simulink model "controllerDevelopment_Simulink"  (R2020b)
settings: Solver=VariableStepAuto  StartTime=0.0  StopTime=10.0  RelTol=1e-3
undefined symbols (not defined in the file or in its folder): K_PID, x_c_0
libraries: cstblocks x6, pid_lib x1
settings Model: Creator=prenk  LastModifiedBy=prenk

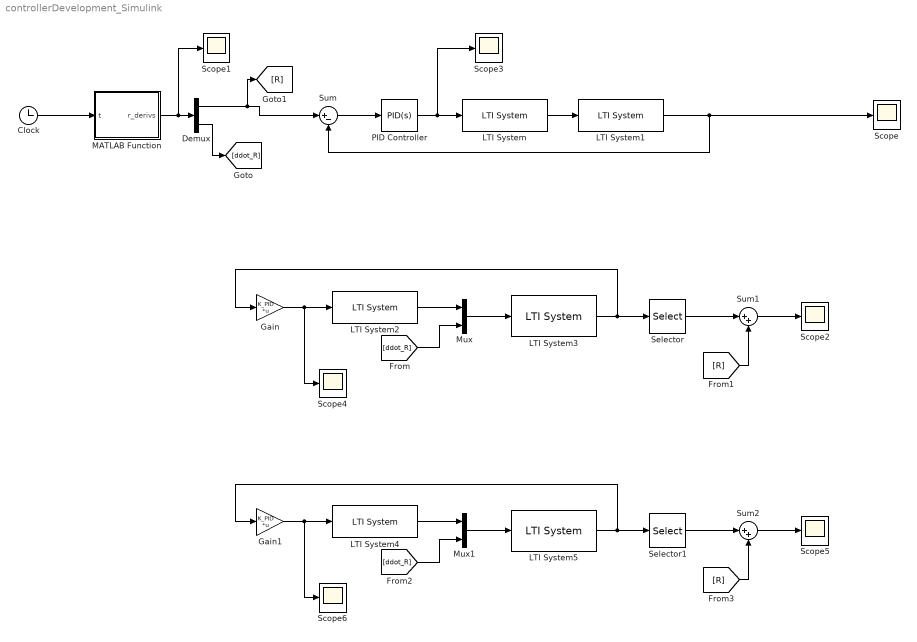
== system controllerDevelopment_Simulink ==
  Clock : Clock
  Demux : Demux  Outputs=2
  Gain : Gain  Gain=K_PID  Multiplication=Matrix(K*u)
  Gain1 : Gain  Gain=K_PID  Multiplication=Matrix(K*u)
  LTI System : cstblocks/LTI System  sys=ssMod_simple_ss  IC=[]
  LTI System1 : cstblocks/LTI System  sys=body  IC=[]
  LTI System2 : cstblocks/LTI System  sys=ssMod_simple_ss  IC=[]
  LTI System3 : cstblocks/LTI System  sys=C_ss  IC=x_c_0
  LTI System4 : cstblocks/LTI System  sys=ssMod_simple_ss  IC=[]
  LTI System5 : cstblocks/LTI System  sys=C_ss  IC=x_c_0
  MATLAB Function : MATLAB Function  TreatAsAtomicUnit=on
  Mux : Mux  Inputs=2
  Mux1 : Mux  Inputs=2
  PID Controller : pid_lib/PID Controller  Controller=PID  Form=Parallel  TimeDomain=Continuous-time  UseExternalTs=off  SampleTime=-1  IntegratorMethod=Forward Euler  FilterMethod=Forward Euler  ControllerParametersSource=internal  P=K_PID(1)  I=K_PID(2)  D=K_PID(3)  UseFilter=on  N=100  TunerSelectOption=Transfer Function Based (PID Tuner App)  InitialConditionSource=internal  InitialConditionForIntegrator=0  InitialConditionForFilter=x_c_0(3)  DifferentiatorICPrevScaledInput=0  ExternalReset=none  TrackingMode=off  Kt=1  LimitOutput=off  SatLimitsSource=internal  UpperSaturationLimit=inf  LowerSaturationLimit=-inf  LinearizeAsGain=on  AntiWindupMode=none  Kb=1  POutMin=[]  POutMax=[]  IOutMin=[]  IOutMax=[]  DOutMin=[]  DOutMax=[]  NOutMin=[]  NOutMax=[]  SumOutMin=[]  SumOutMax=[]  SaturationOutMin=[]  SaturationOutMax=[]  PParamMin=[]  PParamMax=[]  IParamMin=[]  IParamMax=[]  DParamMin=[]  DParamMax=[]  NParamMin=[]  NParamMax=[]  KbParamMin=[]  KbParamMax=[]  KtParamMin=[]  KtParamMax=[]  KbOutMin=[]  KbOutMax=[]  KtOutMin=[]  KtOutMax=[]  IntegratorOutMin=[]  IntegratorOutMax=[]  FilterOutMin=[]  FilterOutMax=[]  SumI1OutMin=[]  SumI1OutMax=[]  SumI2OutMin=[]  SumI2OutMax=[]  SumI3OutMin=[]  SumI3OutMax=[]  SumI4OutMin=[]  SumI4OutMax=[]  SumDOutMin=[]  SumDOutMax=[]  DifferentiatorOutMin=[]  DifferentiatorOutMax=[]  FilterDiffOutCoefMin=[]  FilterDiffOutCoefMax=[]  ReciprocalOutMin=[]  ReciprocalOutMax=[]  SumDenOutMin=[]  SumDenOutMax=[]  SumNumOutMin=[]  SumNumOutMax=[]  DivideOutMin=[]  DivideOutMax=[]  UdiffTsProdOutMin=[]  UdiffTsProdOutMax=[]  NTsProdOutMin=[]  NTsProdOutMax=[]  UintegralTsProdOutMin=[]  UintegralTsProdOutMax=[]  UngainTsProdOutMin=[]  UngainTsProdOutMax=[]  IntegratorContinuousStateAttributes=''  IntegratorStateMustResolveToSignalObject=off  IntegratorRTWStateStorageClass=Auto  FilterContinuousStateAttributes=''  FilterStateMustResolveToSignalObject=off  FilterRTWStateStorageClass=Auto  ParallelPVariant=InternalParameters  IdealPVariant=Disabled  IVariant=InternalParameters  DVariant=InternalParameters  IntegratorVariant=Continuous  SatVariant=Disabled  AWVariant=Passthrough  PCopyVariant=Disabled  TRVariant=Disabled  FdbkBlocksVariant=Forward  IdealPFdbkVariant=Disabled  SatFdbkVariant=Disabled  DerivativeFilterVariant=ContFilter  NVariant=InternalParameters  NCopyVariant=Disabled  FilterICVariant=InternalICsFilter  IntegratorICVariant=InternalICs  ExternalResetVariant=Disabled  TRSumVariant=Passthrough  SumFdbkVariant=Disabled  SumVariant=Sum_PID  TsampFilterVariant=InternalTs  TsampNgainVariant=Passthrough  TsampIntegralVariant=Passthrough  ExternalSaturationOutDataTypeStr=Inherit: Same as second input
  Scope{,1..6} (7 alike) : Scope
  Selector : Selector  InputPortWidth=3  IndexOptions=Index vector (dialog)  Indices=[1]  OutputSizes=1
  Selector1 : Selector  InputPortWidth=3  IndexOptions=Index vector (dialog)  Indices=[1]  OutputSizes=1
  Sum : Sum  Inputs=|+-
  Sum1 : Sum  Inputs=|++
  Sum2 : Sum  Inputs=|++
  wires:
  Demux/1 -> [R], Sum/1
  Sum/1 -> PID Controller/1
  PID Controller/1 -> Scope3/1, LTI System/1
  LTI System/1 -> LTI System1/1
  LTI System1/1 -> Sum/2, Scope/1
  Gain/1 -> Scope4/1, LTI System2/1
  LTI System2/1 -> Mux/1
  Mux/1 -> LTI System3/1
  MATLAB Function/1(r_derivs) -> Scope1/1, Demux/1
  Clock/1 -> MATLAB Function/1(t)
  Demux/2 -> [ddot_R]
  [ddot_R] -> Mux/2
  LTI System3/1 -> Selector/1, Gain/1
  [R] -> Sum1/2
  Sum1/1 -> Scope2/1
  Selector/1 -> Sum1/1
  Selector1/1 -> Sum2/1
  Sum2/1 -> Scope5/1
  [R] -> Sum2/2
  LTI System5/1 -> Gain1/1, Selector1/1
  [ddot_R] -> Mux1/2
  Mux1/1 -> LTI System5/1
  LTI System4/1 -> Mux1/1
  Gain1/1 -> LTI System4/1, Scope6/1

== matlab function controllerDevelopment_Simulink/MATLAB Function ==
  data: t input; r_derivs output
function r_derivs  = fcn(t)
    r1 = -exp(t.*-1.0e+1)+1.0;
    r2 = exp(t.*-1.0e+1).*-1.0e+2;
r_derivs = [r1;r2];
